simulink model "simulation_simple"  (R2024b)
settings: Solver=ode4  StartTime=0.0  StopTime=1500  FixedStep=0.01  RelTol=1e-3
undefined symbols (not defined in the file): at_approach, g_moon, I_total, ka, kr, LLM, masses, q0, r0, rt_approach, rt_breaking, tgo_approach, tgo_breaking, v0, vt_approach, vt_breaking
libraries: simulink x1
settings Model: Creator=gabri  LastModifiedBy=gabri
settings DebuggingCC: UnderSpecifiedDimensionMsg=warning

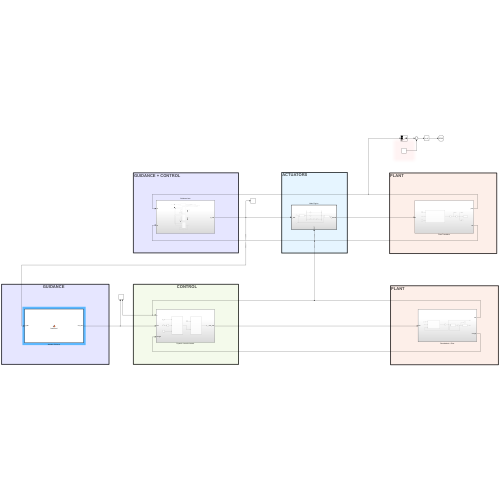
[thumbnail: Simulink's stored preview of the top-level diagram]
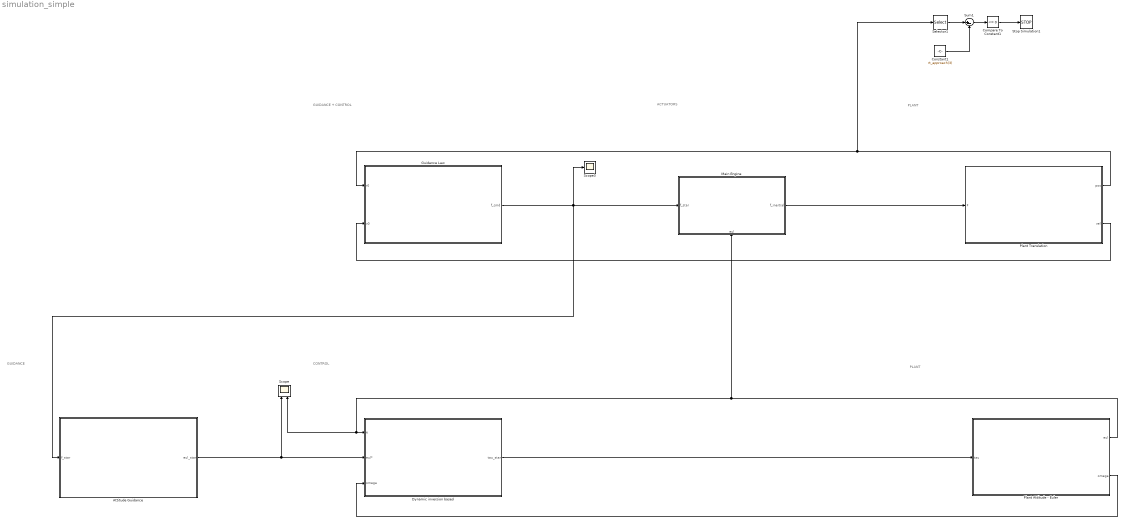
== system simulation_simple ==
  note: PLANT
  note: GUIDANCE
  note: ACTUATORS
  note: GUIDANCE + CONTROL
  note: CONTROL
  note: PLANT
  Attitude Guidance : MATLAB Function  TreatAsAtomicUnit=on
  Compare To Constant1 : simulink/Logic and Bit Operations/Compare To Constant  relop=<=  const=0  OutDataTypeStr=boolean
  Constant1 : Constant  Value=rt_approach(3)
  Dynamic inversion based : Subsystem
  Guidance Law : Subsystem
  Main Engine : Subsystem  TreatAsAtomicUnit=on
      settings: PortSchema="{\"entries\":[{\"content\":{\"sides\":[{\"content\":{\"connectorIds\":[\"In1\"]},\"type\":\"ConnectorPlacement.EquallySpacedRectSide\",\"uuid\":\"1cd70ed7-fffe-4052-be12-d08ec438809a\"},{\"content\":{\"connectorIds\":[\"Out1\"],\"side\":\"RIGHT\"},\"type\":\"ConnectorPlacement.EquallySpacedRectSide\",\"uuid\":\"572c642b-d704-4725-a3d6-bfccbd3ff261\"},{\"content\":{\"side\":\"TOP\"},\"type\":\"ConnectorPlacement.EquallySpacedRectSide\",\"uuid\":\"96cefc9d-2b60-4f61-9fb0-422319e028d1\"},{\"content\":{\"connectorIds\":[\"In2\"],\"side\":\"BOTTOM\"},\"type\":\"ConnectorPlacement.EquallySpacedRectSide\",\"uuid\":\"b823879b-ffc4-494b-bbd8-898eb74a4cd3\"}]},\"type\":\"ConnectorPlacement.EquallySpacedConnector\",\"uuid\":\"14908dc7-5499-48fd-923a-6110af65b868\"}],\"packageUris\":[\"http://schema.mathworks.com/mf0/Connector/R2020b\"],\"version\":\"1.0\"}"
  Plant Attitude - Euler : Subsystem
  Plant Translation : Subsystem
  Scope : Scope  NumInputPorts=2
  Scope3 : Scope
  Selector1 : Selector  InputPortWidth=3  IndexOptions=Index vector (dialog)  Indices=[3]  OutputSizes=1
  Stop Simulation1 : Stop
  Sum1 : Sum  Inputs=|+-
  wires:
  Constant1/1 -> Sum1/2
  Compare To Constant1/1 -> Stop Simulation1/1
  Sum1/1 -> Compare To Constant1/1
  Selector1/1 -> Sum1/1
  Guidance Law/1(f_cmd) -> Scope3/1, Main Engine/1(f_star), Attitude Guidance/1(f_star)
  Attitude Guidance/1(eul_star) -> Dynamic inversion based/2(eul*), Scope/1
  Dynamic inversion based/1(tau_star) -> Plant Attitude - Euler/1(tau)
  Plant Attitude - Euler/1(eul) -> Dynamic inversion based/1(e), Scope/2, Main Engine/2(eul)
  Plant Attitude - Euler/2(omega) -> Dynamic inversion based/3(omega)
  Plant Translation/1(pos) -> Guidance Law/1(r0), Selector1/1
  Main Engine/1(f_inertial) -> Plant Translation/1(F)
  Plant Translation/2(vel) -> Guidance Law/2(v0)

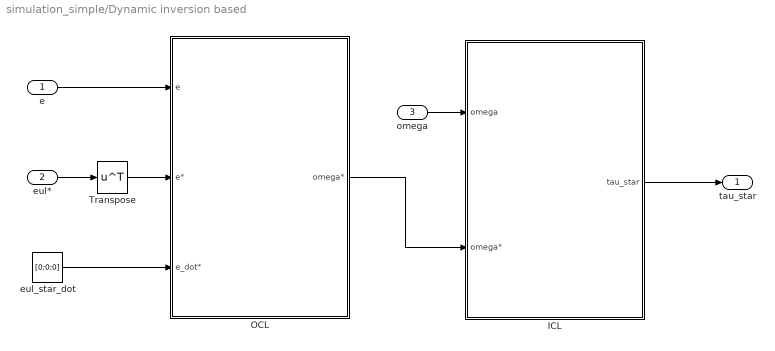
== system simulation_simple/Dynamic inversion based ==
  e : Inport
  eul* : Inport  Port=2
  omega : Inport  Port=3
  ICL : Subsystem  TreatAsAtomicUnit=on
  OCL : Subsystem  TreatAsAtomicUnit=on
  Transpose : Math  Operator=transpose
  eul_star_dot : Constant  Value=[0;0;0]
  tau_star : Outport
  wires:
  eul*/1 -> Transpose/1
  e/1 -> OCL/1(e)
  ICL/1(tau_star) -> tau_star/1
  eul_star_dot/1 -> OCL/3(e_dot*)
  omega/1 -> ICL/1(omega)
  OCL/1(omega*) -> ICL/2(omega*)
  Transpose/1 -> OCL/2(e*)

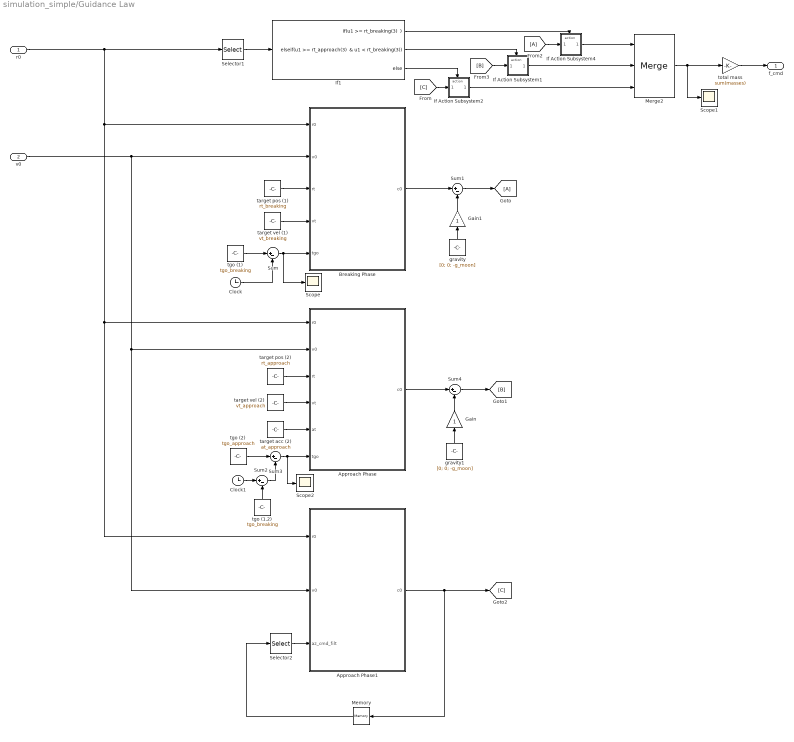
== system simulation_simple/Guidance Law ==
  r0 : Inport
  v0 : Inport  Port=2
  Approach Phase : MATLAB Function  TreatAsAtomicUnit=on
  Approach Phase1 : MATLAB Function  TreatAsAtomicUnit=on
  Breaking Phase : MATLAB Function  TreatAsAtomicUnit=on
  Clock : Clock
  Clock1 : Clock
  From2 : From
  Gain : Gain
  Gain1 : Gain
  Goto : Goto
  If Action Subsystem1 : Subsystem  TreatAsAtomicUnit=on
  If Action Subsystem2 : Subsystem  TreatAsAtomicUnit=on
  If Action Subsystem4 : Subsystem  TreatAsAtomicUnit=on
  If1 : If  IfExpression=u1 >= rt_breaking(3)  ElseIfExpressions="u1 >= rt_approach(3)  & u1 < rt_breaking(3)"
  Memory : Memory
  Merge2 : Merge  Inputs=3
  Scope : Scope
  Scope1 : Scope
  Scope2 : Scope
  Selector1 : Selector  InputPortWidth=3  IndexOptions=Index vector (dialog)  Indices=[3]  OutputSizes=1
  Selector2 : Selector  InputPortWidth=3  IndexOptions=Index vector (dialog)  Indices=[3]  OutputSizes=1
  Sum{,1..4} (5 alike) : Sum  Inputs=|+-
  gravity : Constant  Value=[0; 0; -g_moon]
  gravity1 : Constant  Value=[0; 0; -g_moon]
  target acc (2) : Constant  Value=at_approach
  target pos (1) : Constant  Value=rt_breaking
  target pos (2) : Constant  Value=rt_approach
  target vel (1) : Constant  Value=vt_breaking
  target vel (2) : Constant  Value=vt_approach
  tgo (1) : Constant  Value=tgo_breaking
  tgo (1.2) : Constant  Value=tgo_breaking
  tgo (2) : Constant  Value=tgo_approach
  total mass : Gain  Gain=sum(masses)
  f_cmd : Outport
  wires:
  r0/1 -> Approach Phase1/1(r0), Approach Phase/1(r0), Breaking Phase/1(r0), Selector1/1
  v0/1 -> Approach Phase1/2(v0), Approach Phase/2(v0), Breaking Phase/2(v0)
  target vel (1)/1 -> Breaking Phase/4(vt)
  target pos (1)/1 -> Breaking Phase/3(rt)
  Clock/1 -> Sum/2
  tgo (1)/1 -> Sum/1
  Sum/1 -> Scope/1, Breaking Phase/5(tgo)
  Breaking Phase/1(c0) -> Sum1/1
  gravity/1 -> Gain1/1
  Sum1/1 -> Goto/1
  Sum3/1 -> Approach Phase/6(tgo), Scope2/1
  tgo (2)/1 -> Sum3/1
  Selector1/1 -> If1/1
  target pos (2)/1 -> Approach Phase/3(rt)
  target vel (2)/1 -> Approach Phase/4(vt)
  target acc (2)/1 -> Approach Phase/5(at)
  Sum4/1 -> [B]
  Approach Phase/1(c0) -> Sum4/1
  gravity1/1 -> Gain/1
  [B] -> If Action Subsystem1/1(a_cmd)
  From2/1 -> If Action Subsystem4/1(a_cmd)
  If Action Subsystem1/1(Out1) -> Merge2/2
  If Action Subsystem4/1(Out1) -> Merge2/1
  Merge2/1 -> Scope1/1, total mass/1
  If1/1 -> If Action Subsystem4/Action
  Clock1/1 -> Sum2/1
  Sum2/1 -> Sum3/2
  tgo (1.2)/1 -> Sum2/2
  If1/2 -> If Action Subsystem1/Action
  If1/3 -> If Action Subsystem2/Action
  If Action Subsystem2/1(a_cmd) -> Merge2/3
  Approach Phase1/1(c0) -> Memory/1, [C]
  [C] -> If Action Subsystem2/1(Input)
  Selector2/1 -> Approach Phase1/3(az_cmd_filt)
  Memory/1 -> Selector2/1
  Gain/1 -> Sum4/2
  Gain1/1 -> Sum1/2
  total mass/1 -> f_cmd/1

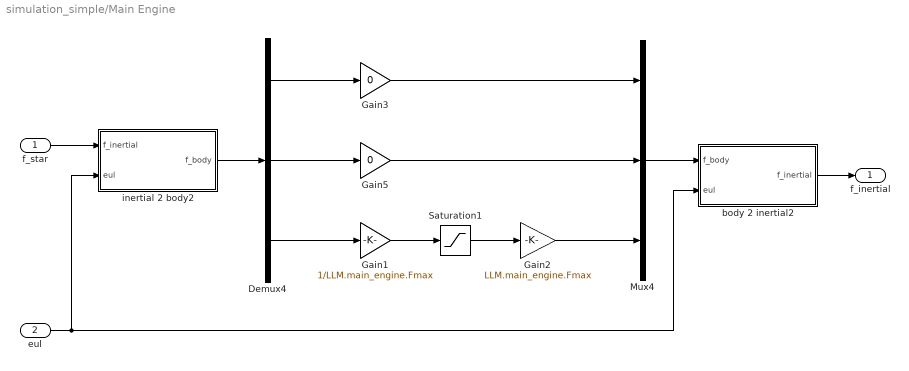
== system simulation_simple/Main Engine ==
  f_star : Inport
  eul : Inport  Port=2
  Demux4 : Demux  Outputs=3
  Gain1 : Gain  Gain=1/LLM.main_engine.Fmax
  Gain2 : Gain  Gain=LLM.main_engine.Fmax
  Gain3 : Gain  Gain=0
  Gain5 : Gain  Gain=0
  Mux4 : Mux  Inputs=3
  Saturation1 : Saturate  UpperLimit=1  LowerLimit=-1
  body 2 inertial2 : MATLAB Function  TreatAsAtomicUnit=on
  inertial 2 body2 : MATLAB Function  TreatAsAtomicUnit=on
  f_inertial : Outport
  wires:
  Demux4/3 -> Gain1/1
  Gain2/1 -> Mux4/3
  Saturation1/1 -> Gain2/1
  Gain1/1 -> Saturation1/1
  Gain3/1 -> Mux4/1
  Demux4/1 -> Gain3/1
  Gain5/1 -> Mux4/2
  Demux4/2 -> Gain5/1
  f_star/1 -> inertial 2 body2/1(f_inertial)
  inertial 2 body2/1(f_body) -> Demux4/1
  Mux4/1 -> body 2 inertial2/1(f_body)
  body 2 inertial2/1(f_inertial) -> f_inertial/1
  eul/1 -> body 2 inertial2/2(eul), inertial 2 body2/2(eul)

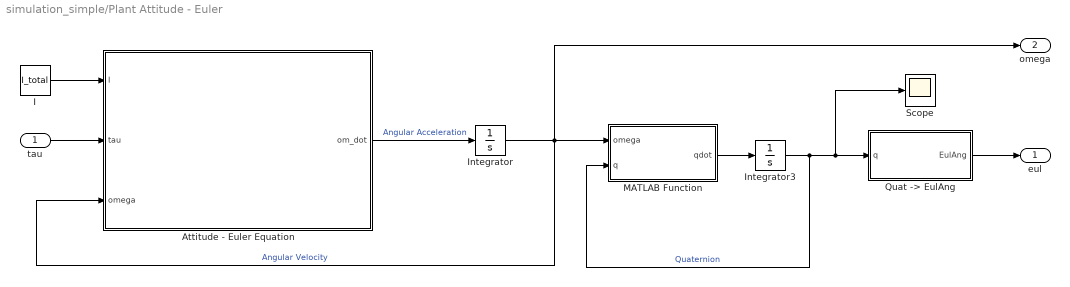
== system simulation_simple/Plant Attitude - Euler ==
  tau : Inport
  Attitude - Euler Equation : MATLAB Function  TreatAsAtomicUnit=on
  I : Constant  Value=I_total
  Integrator : Integrator  InitialCondition=[0; 0; 0]
  Integrator3 : Integrator  InitialCondition=q0'
  MATLAB Function : MATLAB Function  TreatAsAtomicUnit=on
  "Quat -> EulAng" : MATLAB Function  TreatAsAtomicUnit=on
  Scope : Scope
  eul : Outport
  omega : Outport  Port=2
  wires:
  tau/1 -> Attitude - Euler Equation/2(tau)
  Integrator3/1 -> "Quat -> EulAng"/1(q), Scope/1, MATLAB Function/2(q)  "Quaternion"
  MATLAB Function/1(qdot) -> Integrator3/1
  Integrator/1 -> omega/1, MATLAB Function/1(omega), Attitude - Euler Equation/3(omega)  "Angular Velocity"
  I/1 -> Attitude - Euler Equation/1(I)
  "Quat -> EulAng"/1(EulAng) -> eul/1
  Attitude - Euler Equation/1(om_dot) -> Integrator/1  "Angular Acceleration"

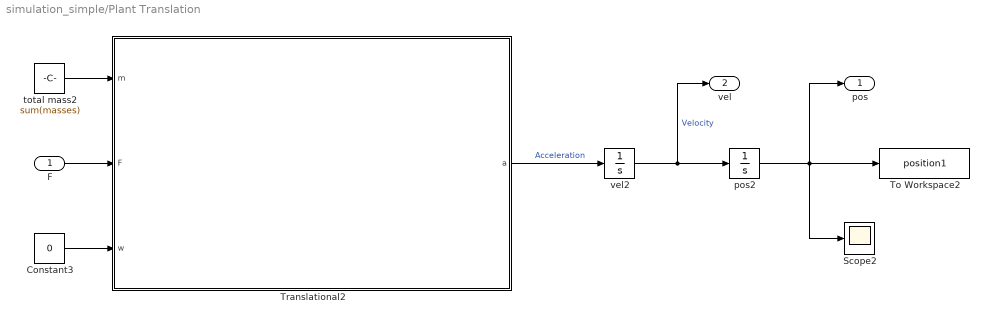
== system simulation_simple/Plant Translation ==
  F : Inport
  Constant3 : Constant  Value=0
  Scope2 : Scope
  To Workspace2 : ToWorkspace  VariableName=position1  SampleTime=-1
  Translational2 : MATLAB Function  TreatAsAtomicUnit=on
  pos2 : Integrator  InitialCondition=r0
  total mass2 : Constant  Value=sum(masses)
  vel2 : Integrator  InitialCondition=v0
  pos : Outport
  vel : Outport  Port=2
  wires:
  Translational2/1(a) -> vel2/1  "Acceleration"
  total mass2/1 -> Translational2/1(m)
  pos2/1 -> Scope2/1, pos/1, To Workspace2/1
  Constant3/1 -> Translational2/3(w)
  F/1 -> Translational2/2(F)
  vel2/1 -> vel/1, pos2/1  "Velocity"

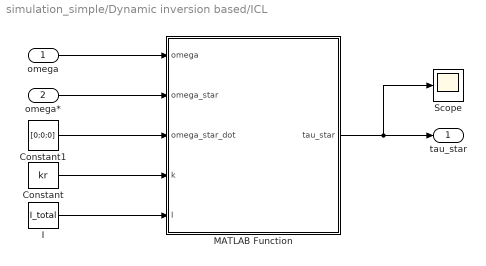
== system simulation_simple/Dynamic inversion based/ICL ==
  omega : Inport
  omega* : Inport  Port=2
  Constant : Constant  Value=kr
  Constant1 : Constant  Value=[0;0;0]
  I : Constant  Value=I_total
  MATLAB Function : MATLAB Function  TreatAsAtomicUnit=on
  Scope : Scope
  tau_star : Outport
  wires:
  omega/1 -> MATLAB Function/1(omega)
  MATLAB Function/1(tau_star) -> Scope/1, tau_star/1
  omega*/1 -> MATLAB Function/2(omega_star)
  Constant/1 -> MATLAB Function/4(k)
  I/1 -> MATLAB Function/5(I)
  Constant1/1 -> MATLAB Function/3(omega_star_dot)

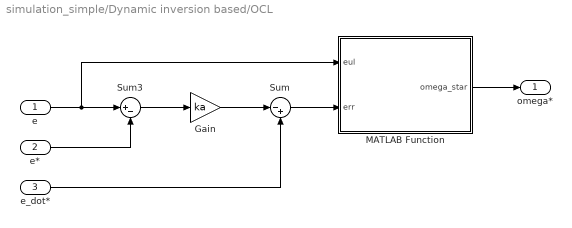
== system simulation_simple/Dynamic inversion based/OCL ==
  e : Inport
  e* : Inport  Port=2
  e_dot* : Inport  Port=3
  Gain : Gain  Gain=ka
  MATLAB Function : MATLAB Function  TreatAsAtomicUnit=on
  Sum : Sum  Inputs=|-+
  Sum3 : Sum  Inputs=|+-
  omega* : Outport
  wires:
  e/1 -> MATLAB Function/1(eul), Sum3/1
  e*/1 -> Sum3/2
  Sum3/1 -> Gain/1
  MATLAB Function/1(omega_star) -> omega*/1
  e_dot*/1 -> Sum/2
  Gain/1 -> Sum/1
  Sum/1 -> MATLAB Function/2(err)

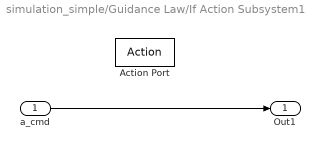
== system simulation_simple/Guidance Law/If Action Subsystem1 ==
  a_cmd : Inport
  Action Port : ActionPort  ActionPortLabel=elseif(..)
  Out1 : Outport
  wires:
  a_cmd/1 -> Out1/1

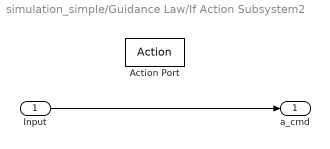
== system simulation_simple/Guidance Law/If Action Subsystem2 ==
  Input : Inport
  Action Port : ActionPort  ActionPortLabel=else
  a_cmd : Outport
  wires:
  Input/1 -> a_cmd/1

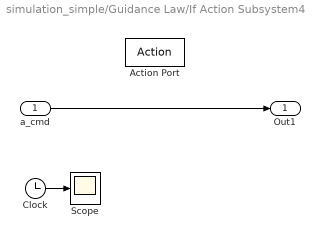
== system simulation_simple/Guidance Law/If Action Subsystem4 ==
  a_cmd : Inport
  Action Port : ActionPort  ActionPortLabel="if(u1 >= rt_breaking(3)  )"
  Clock : Clock
  Scope : Scope
  Out1 : Outport
  wires:
  a_cmd/1 -> Out1/1
  Clock/1 -> Scope/1

== matlab function simulation_simple/Plant Attitude - Euler/MATLAB Function ==
  data: omega input; qdot output; q input
function qdot = fcn(omega,q)

Omega = [0 -omega(1) -omega(2) -omega(3);
         omega(1) 0 omega(3) omega(2);
         omega(2) omega(3) 0 omega(1);
         omega(3) omega(2) omega(1) 0];

q0 = q(1);
q1 = q(2);
q2 = q(3);
q3 = q(4);

qdot = 0.5*Omega*[q0 q1 q2 q3]';

== matlab function simulation_simple/Plant Attitude - Euler/Quat -> EulAng ==
  data: q input; EulAng output
function EulAng = fcn(q)

    qs = q(1); qx = q(2); qy = q(3); qz = q(4);
    
    EulAng = [-atan2(2*(-qs*qx+qy*qz), -qx^2-qy^2+qz^2+qs^2);
              atan2(2*(qz*qx+qy*qs), (1-(2*(qz*qx+qy*qs))^2)^.5); %asin(2*(qz*qx+qyqs));
              -atan2(2*(-qs*qz+qx*qy), qx^2-qy^2-qz^2+qs^2)];

end

== matlab function simulation_simple/Attitude Guidance ==
  data: f_star input; eul_star output
function eul_star = force2eul(f_star)

    R1 = @(bank)  [cos(bank) sin(bank) 0; -sin(bank) cos(bank) 0; 0 0 1];
    R2 = @(pitch) [sin(pitch) 0 -cos(pitch); 0 1 0; cos(pitch) 0 sin(pitch)];
    
    bank = atan2(f_star(2,:),f_star(1,:));
    f_cmd_rot = R1(bank)*f_star;
    pitch = atan2(f_cmd_rot(3,:),f_cmd_rot(1,:));
    R = R2(pitch)*R1(bank);
    eul_star = rotm2eul(R,'ZYX');
    eulx = eul_star(3); euly = eul_star(2); eulz = eul_star(1);

    % eul_star = zeros(3,1);
    eul_star(1) = eulx; eul_star(2) = euly; eul_star(3) = eulz;
        
end

== matlab function simulation_simple/Guidance Law/Approach Phase ==
  data: r0 input; c0 output; v0 input; rt input; vt input; at input; tgo input
function c0 = approach_coeffs(r0,v0,rt,vt,at,tgo)

    c0 = at - 6*(vt+v0)/tgo + 12*(rt - r0)/(tgo^2);
    if tgo<1
        tgo = 1;
        c0 = [0; 0; -1.63];
    end

end

== matlab function simulation_simple/Guidance Law/Approach Phase1 ==
  data: r0 input; c0 output; v0 input; az_cmd_filt input
function c0 = approach_coeffs(r0,v0,az_cmd_filt)
    
    g_moon  = 1.62;
    az3_cmd = 1.2*g_moon;

    clip = @(u,umin,umax) max(min(u,umax),umin);

    if ~exist('Kxy','var'),      Kxy = 0.8; end
    if ~exist('ax_max','var'),   ax_max = 2.0; end
    if ~exist('ay_max','var'),   ay_max = 2.0; end
    if ~exist('daz_max','var'),  daz_max = 0.6*g_moon; end
    if ~exist('az_cmd_filt','var'), az_cmd_filt = az3_cmd; end
    
    v_td   = -0.1;                 % m/s target at impact
    az_nom = az3_cmd;              % m/s^2 (1.2 g_moon)
    az_max = az_nom + daz_max;     % thrust bound
    a_up_max = max(az_max - g_moon, 0.1);  % net braking capability
    alpha_f  = 0.6;                % smoothing 0..1
    
    % (2) DIVERT table (from your table)
    divert_D   = [25   50    75   100   125   150];      % m
    divert_dT  = [-0.9 -0.6  4.0   8.3   11.1  15.4];    % s
    divert_dDV = [-0.9  0.6  8.2  15.5   20.3  27.4];    % m/s (info)
    
    % Additional remaining time (decreases over time)
    dT_hold = 0;    % s
    dDV_est = 0;    % m/s (optional, for log)
    
    % ================== 1) Horizontal correctors ==================
    if r0(3) > 50
        vx_lim = 10; vy_lim = 10;      % limits under 50 m
        ax_cmd = (abs(v0(1))>vx_lim) * (-Kxy*(abs(v0(1))-vx_lim)*sign(v0(1)));
        ay_cmd = (abs(v0(2))>vy_lim) * (-Kxy*(abs(v0(2))-vy_lim)*sign(v0(2)));
    else
        band = 0.1;                    % deadband ±0.1 m/s under 10 m
        ax_cmd = (v0(1)> band)*(-Kxy*(v0(1)-band)) + (v0(1)<-band)*(-Kxy*(v0(1)+band));
        ay_cmd = (v0(2)> band)*(-Kxy*(v0(2)-band)) + (v0(2)<-band)*(-Kxy*(v0(2)+band));
    end
    ax_cmd = clip(ax_cmd,-ax_max,ax_max);
    ay_cmd = clip(ay_cmd,-ay_max,ay_max);

    % ================== 2) DIVERT management (lateral distance) ========
    D = hypot(r0(1),r0(2));                                   % m
    dT_target = interp1(divert_D, divert_dT, D, 'linear','extrap');
    dDV_target = interp1(divert_D, divert_dDV, D, 'linear','extrap');

    % Never shorten the descent: keep only ΔT>0
    dT_target = max(0, dT_target);
    % Keep the maximum time need observed and consume it progressively
    dT_hold = max(dT_hold, dT_target);
    dDV_est = max(dDV_est, max(0,dDV_target));       % info (not used in loop)

    % Rough estimate of remaining time (used to normalize stretching)
    tgo_est = r0(3) / max(0.5, -v0(3) + 0.1);               % s, robust if vz≈0
    slow_factor = 1 + min(0.8, dT_hold / max(5, tgo_est));   % ≤ +80% on τ

    % ================== 3) Vertical profile v_ref(z) ==================
    v_env = -sqrt(max(v_td^2 + 2*a_up_max*max(r0(3),0), 0));   % stoppable envelope
    if     r0(3) > 200, v_cap = v_env;
    elseif r0(3) > 50,  v_cap = max(v_env, -2);   % intermediate speed limit
    elseif r0(3) > 5,   v_cap = max(v_env, -1);
    else            v_cap = max(v_env, v_td); % converge to -0.2 m/s
    end
    v_ref = v_cap;

    % Base time constant (tighter near ground), then “stretched” by DIVERT
    if     r0(3) > 200, tau = 12.0;
    elseif r0(3) > 100, tau = 6.0;
    elseif r0(3) > 50,  tau = 4.0;
    elseif r0(3) > 20,  tau = 2.0;
    elseif r0(3) > 5,  tau = 1.5;
    else            tau = 2;
    end
    tau = tau * slow_factor;     % <<< buy time for DIVERT

    % Desired net acceleration & commanded thrust
    a_net_des = (v_ref - v0(3))/tau;                   % m/s^2
    az_cmd_raw = g_moon + a_net_des;                % m->thrust
    az_cmd_raw = clip(az_cmd_raw, 0, az_max);
    az_cmd = alpha_f*az_cmd_filt + (1-alpha_f)*az_cmd_raw;
    
    c0 = [ax_cmd; ay_cmd; az_cmd];
    
end

== matlab function simulation_simple/Guidance Law/Breaking Phase ==
  data: r0 input; c0 output; v0 input; rt input; vt input; tgo input
function c0 = braking_coeffs(r0, v0, rt, vt, tgo)
    
    c0 = (-2*(vt+2*v0))/tgo + 6*(rt - r0)/(tgo^2);
    if tgo<0.5
        c0 = [0; 0; -1.63];
    end

end

== matlab function simulation_simple/Plant Translation/Translational2 ==
  data: m input; F input; a output; w input
function a = translation(m, F, w)

% lunar gravity in inertial frame (verso -Z)
gL = 1.622;
g = [0; 0; -gL];

a = F./m + g;

end

== matlab function simulation_simple/Main Engine/body 2 inertial2 ==
  data: f_body input; eul input; f_inertial output
function f_inertial = fcn(f_body,eul)

% Using quaternions
% q0 = q(1);
% q1 = q(2);
% q2 = q(3);
% q3 = q(4);
% R = [q0^2+q1^2-q2^2-q3^2 2*(q1*q2-q0*q3) 2*(q1*q3+q0*q2);
%      2*(q1*q2+q0*q3) q0^2-q1^2+q2^2-q3^2 2*(q2*q3-q0*q1);
%      2*(q1*q3-q0*q2) 2*(q2*q3+q0*q1) q0^2-q1^2-q2^2+q3^2];


% Using euler angles (ZYX)
% eul(1) rotation around x
% eul(2) rotation around y'
% eul(3) rotation around z''
Rx = @(thx) [1 0 0; 0 cos(thx) -sin(thx); 0 sin(thx) cos(thx)];
Ry = @(thy) [cos(thy) 0 sin(thy); 0 1 0; -sin(thy) 0 cos(thy)];
Rz = @(thz) [cos(thz) -sin(thz) 0; sin(thz) cos(thz) 0; 0 0 1];
R = Rz(eul(3))*Ry(eul(2))*Rx(eul(1));
f_inertial = R'*f_body;

== matlab function simulation_simple/Main Engine/inertial 2 body2 ==
  data: f_inertial input; eul input; f_body output
function f_body = fcn(f_inertial,eul)

% Using quaternions
% q0 = q(1);
% q1 = q(2);
% q2 = q(3);
% q3 = q(4);
% R = [q0^2+q1^2-q2^2-q3^2 2*(q1*q2-q0*q3) 2*(q1*q3+q0*q2);
%      2*(q1*q2+q0*q3) q0^2-q1^2+q2^2-q3^2 2*(q2*q3-q0*q1);
%      2*(q1*q3-q0*q2) 2*(q2*q3+q0*q1) q0^2-q1^2-q2^2+q3^2];


% Using euler angles (ZYX)
% eul(1) rotation around x
% eul(2) rotation around y'
% eul(3) rotation around z''
Rx = @(thx) [1 0 0; 0 cos(thx) -sin(thx); 0 sin(thx) cos(thx)];
Ry = @(thy) [cos(thy) 0 sin(thy); 0 1 0; -sin(thy) 0 cos(thy)];
Rz = @(thz) [cos(thz) -sin(thz) 0; sin(thz) cos(thz) 0; 0 0 1];
R = Rz(eul(3))*Ry(eul(2))*Rx(eul(1));
f_body = R*f_inertial;

== matlab function simulation_simple/Dynamic inversion based/ICL/MATLAB Function ==
  data: omega input; tau_star output; omega_star input; omega_star_dot input; k input; I input
function tau_star = fcn(omega, omega_star, omega_star_dot, k ,I)
    
    tau_max = 4e3;
    tau_star = I*(omega_star_dot-k.*(omega-omega_star)) + [(I(3)-I(2))*omega(2)*omega(3); (I(1)-I(3))*omega(1)*omega(3); (I(2)-I(1))*omega(1)*omega(2)];
    tau_star = min(max(tau_star, -tau_max), tau_max);

end

== matlab function simulation_simple/Dynamic inversion based/OCL/MATLAB Function ==
  data: eul input; omega_star output; err input
function omega_star = fcn(eul, err)
    
    err = wrapToPi(err);
    T = [1  0 -sin(eul(2));
         0  cos(eul(1)) sin(eul(1))*cos(eul(2));
         0 -sin(eul(1)) cos(eul(1))*cos(eul(2))];
    if err(2)>0
        a=1;
    end
    omega_star = T*err;
    omega_star = max(min(omega_star, 0.7), -0.7);

end

== matlab function simulation_simple/Plant Attitude - Euler/Attitude - Euler Equation ==
  data: I input; om_dot output; tau input; omega input
function om_dot = rotation(I, tau, omega)
    
    om_dot = inv(I)*(tau-cross(omega,I*omega));

end
